simulink model "Parking_Assist"  (R2025a)
settings: Solver=VariableStepAuto  StartTime=0.0  StopTime=30  RelTol=1e-3
settings Model: Creator=Rudransh  LastModifiedBy=Rudransh

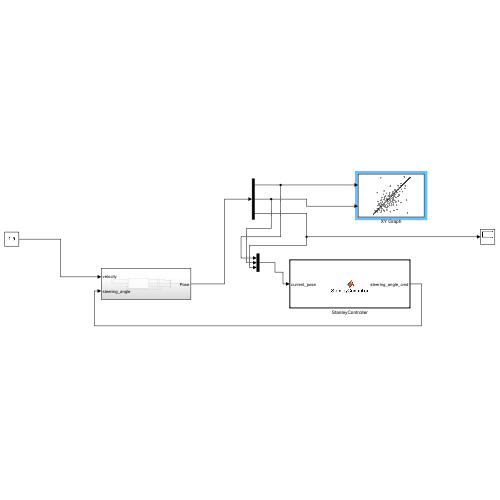
[thumbnail: Simulink's stored preview of the top-level diagram]
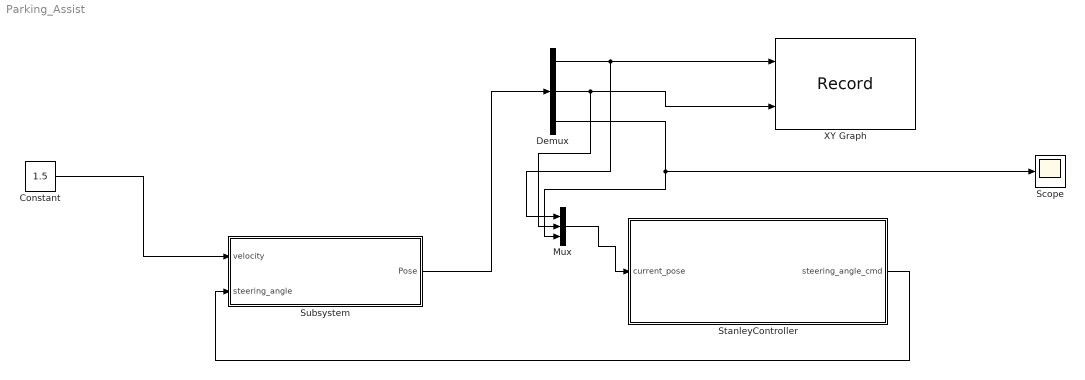
== system Parking_Assist ==
  Constant : Constant  Value=1.5
  Demux : Demux  Outputs=3
  Mux : Mux  Inputs=3
  Scope : Scope
      settings: Title=SteeringRotation  ActiveDisplayYMinimum=-0.0820382939889809  ActiveDisplayYMaximum=0.73834464590082816
  StanleyController : MATLAB Function  TreatAsAtomicUnit=on
  Subsystem : Subsystem
  XY Graph : Record  NumPorts=2.0  FileSettingsInternal="{\"entries\":[{\"content\":{\"excelSettings\":{\"content\":{},\"type\":\"Streamout.ExcelSettings\"},\"parquetSettings\":{\"content\":{},\"type\":\"Streamout.ParquetSettings\"}},\"type\":\"Streamout.FileSettingStorage\",\"uuid\":\"\"}],\"packageUris\":[\"http:\\/\\/schema.mathworks.com\\/mf0\\/streamout_blocks\\/R2020a\"],\"version\":\"1.0\"}"  FrameSettings=[0, 0]  Layout=[1 1]  SignalsInternal="{\"entries\":[{\"content\":{\"signals\":[{\"content\":{\"blockPath\":[],\"dimensions\":[1,1],\"domain\":\"\",\"lineColor\":\"#a2142f\",\"plots\":[ 1 ],\"port\":1,\"sid\":[\"\"],\"signalID\":1,\"signalName\":\"Demux:1\"},\"type\":\"RecordBlkView.Signal\",\"uuid\":\"\"},{\"content\":{\"blockPath\":[],\"dimensions\":[1,1],\"domain\":\"\",\"lineColor\":\"#139fff\",\"plots\":[ 1 ],\"port\":2,\"sid\":[\"\"],\"signalID\":2,\"signalName\":\"Demux:2\"},\"type\":\"RecordBlkView.Signal\",\"uuid\":\"\"}]},\"type\":\"RecordBlkView.InputSignals\",\"uuid\":\"\"}],\"packageUris\":[\"http:\\/\\/schema.mathworks.com\\/mf0\\/streamout_blocks\\/R2020a\"],\"version\":\"1.0\"}"  VisualizationBindings="{\"xyplotplugin\":{\"info\":[{\"series\":[{\"bindingParametersList\":[{\"parameter\":\"X-Axis\",\"signalID\":1,\"signalName\":\"Demux:1\"},{\"parameter\":\"Y-Axis\",\"signalID\":2,\"signalName\":\"Demux:2\"}],\"seriesID\":0}],\"subplotID\":1}]}}"  CompatibilityTag=XY
  wires:
  Subsystem/1(Pose) -> Demux/1
  StanleyController/1(steering_angle_cmd) -> Subsystem/2(steering_angle)
  Constant/1 -> Subsystem/1(velocity)
  Demux/1 -> Mux/1, XY Graph/1
  Demux/2 -> Mux/2, XY Graph/2
  Demux/3 -> Mux/3, Scope/1
  Mux/1 -> StanleyController/1(current_pose)

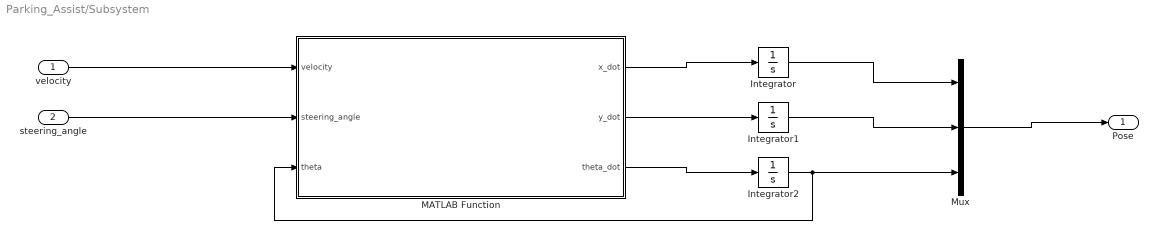
== system Parking_Assist/Subsystem ==
  velocity : Inport
  steering_angle : Inport  Port=2
  Integrator : Integrator
  Integrator1 : Integrator
  Integrator2 : Integrator
  MATLAB Function : MATLAB Function  TreatAsAtomicUnit=on
  Mux : Mux  Inputs=3
  Pose : Outport
  wires:
  MATLAB Function/3(theta_dot) -> Integrator2/1
  MATLAB Function/2(y_dot) -> Integrator1/1
  MATLAB Function/1(x_dot) -> Integrator/1
  Integrator2/1 -> MATLAB Function/3(theta), Mux/3
  Integrator1/1 -> Mux/2
  Integrator/1 -> Mux/1
  Mux/1 -> Pose/1
  steering_angle/1 -> MATLAB Function/2(steering_angle)
  velocity/1 -> MATLAB Function/1(velocity)

== matlab function Parking_Assist/StanleyController ==
  data: steering_angle_cmd output size=1; current_pose input size=[1 3]
function steering_angle_cmd = StanleyController(current_pose)

% Use a persistent variable to load the path only once
persistent path;
if isempty(path)
    % Load path data from the .mat file
    path_data = load('parkingPath.mat');
    path = path_data.path_waypoints;
end

% Controller parameters
k = 0.5; % Cross-track error gain
velocity = 1.5; % Assume constant low speed for parking (m/s)

% Extract current vehicle state
x = current_pose(1);
y = current_pose(2);
theta = current_pose(3);

% --- Find the closest point on the path ---
[~, nearest_idx] = min(sqrt((path(:,1) - x).^2 + (path(:,2) - y).^2));

% Get reference pose from the path
x_ref = path(nearest_idx, 1);
y_ref = path(nearest_idx, 2);
theta_ref = path(nearest_idx, 3);

% --- Calculate Errors ---
% 1. Heading Error
heading_error = theta_ref - theta;
heading_error = atan2(sin(heading_error), cos(heading_error));

% 2. Cross-Track Error
cross_track_error = (x - x_ref)*cos(theta_ref + pi/2) + (y - y_ref)*sin(theta_ref + pi/2);

% --- Stanley Law Steering Command ---
steering_angle_cmd = heading_error + atan2(k * cross_track_error, velocity);

% --- Saturate the steering angle ---
max_steer = 0.6; % radians (~35 degrees)
if abs(steering_angle_cmd) > max_steer
    steering_angle_cmd = sign(steering_angle_cmd) * max_steer;
end

end

== matlab function Parking_Assist/Subsystem/MATLAB Function ==
  data: velocity input; x_dot output; steering_angle input; theta input; y_dot output; theta_dot output
function [x_dot, y_dot, theta_dot] = KinematicEquations(velocity, steering_angle, theta)
% This function calculates the RATES of change, not the position.
L = 2.8; % Wheelbase
x_dot = velocity * cos(theta);
y_dot = velocity * sin(theta);
theta_dot = (velocity / L) * tan(steering_angle);
end
